simulink subsystem "bh_COMPONENT_model_7dof_car_SCAPE"  (R2022b)
settings: Solver=VariableStepAuto  StartTime=0.0  StopTime=10.0  RelTol=1e-3
model mask{L_b=0, L_f=0, L_R=0, L_L=0, m_c=0, I_cZ=0, I_cX=0, m_bR=0, m_fR=0, m_bL=0, m_fL=0, k_bR=0, k_fR=0, k_bL=0, k_fL=0, k_bRG=0, k_fRG=0, k_bLG=0, k_fLG=0, c_bR=0, c_fR=0, c_bL=0, c_fL=0, c_bRG=0, c_fRG=0, c_bLG=0, c_fLG=0, IC_pos=zeros(7,1), IC_vel=zeros(7,1)}
  mask prompts: L_b "L_b   (m)"; L_f "L_f   (m)"; L_R "L_R   (m)"; L_L "L_L   (m)"; m_c "m_c     (kg)"; I_cZ "I_cZ      (kg.m^2)"; I_cX "I_cX      (kg.m2)"; m_bR "m_bR   (kg)"; m_fR "m_fR    (kg)"; m_bL "m_bL   (kg)"; m_fL "m_fL    (kg)"; k_bR "k_bR   (N/m)"; k_fR "k_fR   (N/m)"; k_bL "k_bL   (N/m)"; k_fL "k_fL    (N/m)"; k_bRG "k_bRG   (N/m)"; k_fRG "k_fRG   (N/m)"; k_bLG "k_bLG   (N/m)"; k_fLG "k_fLG    (N/m)"; c_bR "c_bR  (N.s/m)"; c_fR "c_fR  (N.s/m)"; c_bL "c_bL  (N.s/m)"; c_fL "c_fL  (N.s/m)"; c_bRG "c_bRG  (N.s/m)"; c_fRG "c_fRG  (N.s/m)"; c_bLG "c_bLG  (N.s/m)"; c_fLG "c_fLG  (N.s/m)"
undefined symbols (not defined in the file): X, Y, Z
libraries: sm_lib x37, fl_lib x32, nesl_utility x14
settings Model: Creator=bhorton  LastModifiedBy=bhorton
settings DebuggingCC: UnconnectedInputMsg=warning  UnconnectedOutputMsg=warning  UnconnectedLineMsg=warning
settings ModelReferenceCC: EnableRefExpFcnMdlSchedulingChecks=on
settings RTWCC: DLArmComputeVersion=19.05

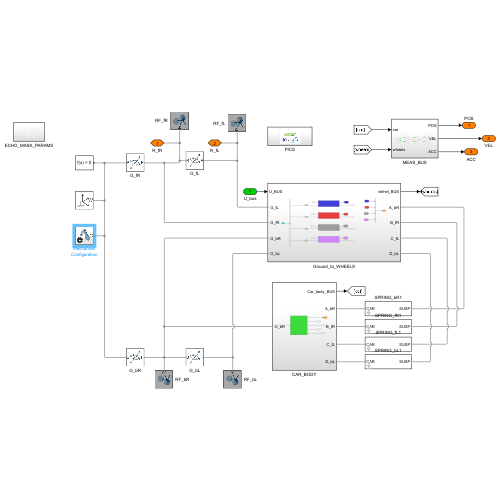
[thumbnail: Simulink's stored preview of the top-level diagram]
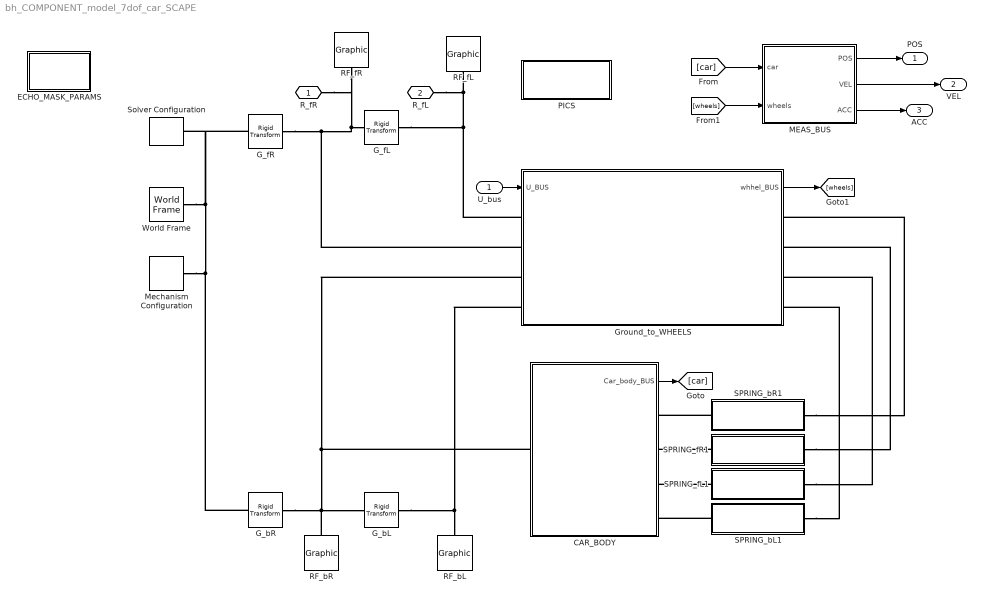
== system bh_COMPONENT_model_7dof_car_SCAPE ==
  U_bus : Inport
  CAR_BODY : Subsystem
  ECHO_MASK_PARAMS : Subsystem
  G_bL : sm_lib/Frames and Transforms/Rigid Transform  TranslationMethod=StandardAxis  TranslationStandardOffset=(L_L + L_R)  TranslationLengthUnit=m  TranslationStandardAxis=-Z  TranslationCartesianOffset=[0 0 0]  TranslationROffset=0  TranslationROffsetUnits=m  TranslationZOffset=0  TranslationZOffsetUnits=m  TranslationThetaOffset=0  TranslationThetaOffsetUnits=deg  RotationMethod=None  RotationAngleUnits=deg  RotationStandardAxis=+Z  RotationAngle=0.0  RotationArbitraryAxis=[0 0 1]  FollAlignAxisA=+X  BaseAlignAxisA=+Y  FollAlignAxisB=+Y  BaseAlignAxisB=+Z  RotationSequenceAxes=FollowerAxes  RotationSequence=XYX  RotationSequenceAngles=[0 0 0]  RotationSequenceAnglesUnits=deg  RotationMatrix=[1 0 0; 0 1 0; 0 0 1]  Quaternion=[1 0 0 0]
  G_bR : sm_lib/Frames and Transforms/Rigid Transform  TranslationMethod=None  TranslationStandardOffset=0  TranslationLengthUnit=m  TranslationStandardAxis=-X  TranslationCartesianOffset=[0 0 0]  TranslationROffset=0  TranslationROffsetUnits=m  TranslationZOffset=0  TranslationZOffsetUnits=m  TranslationThetaOffset=0  TranslationThetaOffsetUnits=deg  RotationMethod=None  RotationAngleUnits=deg  RotationStandardAxis=+Z  RotationAngle=0.0  RotationArbitraryAxis=[0 0 1]  FollAlignAxisA=+X  BaseAlignAxisA=+Y  FollAlignAxisB=+Y  BaseAlignAxisB=+Z  RotationSequenceAxes=FollowerAxes  RotationSequence=XYX  RotationSequenceAngles=[0 0 0]  RotationSequenceAnglesUnits=deg  RotationMatrix=[1 0 0; 0 1 0; 0 0 1]  Quaternion=[1 0 0 0]
  G_fL : sm_lib/Frames and Transforms/Rigid Transform  TranslationMethod=StandardAxis  TranslationStandardOffset=(L_L + L_R)  TranslationLengthUnit=m  TranslationStandardAxis=-Z  TranslationCartesianOffset=[0 0 0]  TranslationROffset=0  TranslationROffsetUnits=m  TranslationZOffset=0  TranslationZOffsetUnits=m  TranslationThetaOffset=0  TranslationThetaOffsetUnits=deg  RotationMethod=None  RotationAngleUnits=deg  RotationStandardAxis=+Z  RotationAngle=0.0  RotationArbitraryAxis=[0 0 1]  FollAlignAxisA=+X  BaseAlignAxisA=+Y  FollAlignAxisB=+Y  BaseAlignAxisB=+Z  RotationSequenceAxes=FollowerAxes  RotationSequence=XYX  RotationSequenceAngles=[0 0 0]  RotationSequenceAnglesUnits=deg  RotationMatrix=[1 0 0; 0 1 0; 0 0 1]  Quaternion=[1 0 0 0]
  G_fR : sm_lib/Frames and Transforms/Rigid Transform  TranslationMethod=StandardAxis  TranslationStandardOffset=(L_b + L_f)  TranslationLengthUnit=m  TranslationStandardAxis=+X  TranslationCartesianOffset=[0 0 0]  TranslationROffset=0  TranslationROffsetUnits=m  TranslationZOffset=0  TranslationZOffsetUnits=m  TranslationThetaOffset=0  TranslationThetaOffsetUnits=deg  RotationMethod=None  RotationAngleUnits=deg  RotationStandardAxis=+Z  RotationAngle=0.0  RotationArbitraryAxis=[0 0 1]  FollAlignAxisA=+X  BaseAlignAxisA=+Y  FollAlignAxisB=+Y  BaseAlignAxisB=+Z  RotationSequenceAxes=FollowerAxes  RotationSequence=XYX  RotationSequenceAngles=[0 0 0]  RotationSequenceAnglesUnits=deg  RotationMatrix=[1 0 0; 0 1 0; 0 0 1]  Quaternion=[1 0 0 0]
  Ground_to_WHEELS : Subsystem
  MEAS_BUS : Subsystem
  Mechanism Configuration : sm_lib/Utilities/Mechanism Configuration  UniformGravity=Constant  GravityVector=[0 0 0]  GravityUnits=m/s^2  LinearizationDelta=0.001  JointModeTransitionNonlinearIterations=2
  PICS : Subsystem
  RF_bL : sm_lib/Body Elements/Graphic  GraphicType=Marker  MarkerShape=Frame  MarkerSize=30  GraphicVisPropType=SimpleVisualProperties  GraphicDiffuseColor=[0.0 0.0 0.0]  GraphicSpecularColor=[0.5 0.5 0.5 1.0]  GraphicAmbientColor=[0.15 0.15 0.15 1.0]  GraphicEmissiveColor=[0.0 0.0 0.0 1.0]  GraphicShininess=75  GraphicOpacity=1.0
  RF_bR : sm_lib/Body Elements/Graphic  GraphicType=Marker  MarkerShape=Frame  MarkerSize=30  GraphicVisPropType=SimpleVisualProperties  GraphicDiffuseColor=[0.0 0.0 0.0]  GraphicSpecularColor=[0.5 0.5 0.5 1.0]  GraphicAmbientColor=[0.15 0.15 0.15 1.0]  GraphicEmissiveColor=[0.0 0.0 0.0 1.0]  GraphicShininess=75  GraphicOpacity=1.0
  RF_fL : sm_lib/Body Elements/Graphic  GraphicType=Marker  MarkerShape=Frame  MarkerSize=30  GraphicVisPropType=SimpleVisualProperties  GraphicDiffuseColor=[0.0 0.0 0.0]  GraphicSpecularColor=[0.5 0.5 0.5 1.0]  GraphicAmbientColor=[0.15 0.15 0.15 1.0]  GraphicEmissiveColor=[0.0 0.0 0.0 1.0]  GraphicShininess=75  GraphicOpacity=1.0
  RF_fR : sm_lib/Body Elements/Graphic  GraphicType=Marker  MarkerShape=Frame  MarkerSize=30  GraphicVisPropType=SimpleVisualProperties  GraphicDiffuseColor=[0.0 0.0 0.0]  GraphicSpecularColor=[0.5 0.5 0.5 1.0]  GraphicAmbientColor=[0.15 0.15 0.15 1.0]  GraphicEmissiveColor=[0.0 0.0 0.0 1.0]  GraphicShininess=75  GraphicOpacity=1.0
  SPRING_bL1 : Subsystem  mask{c=c_bL, k=k_bL, EQ_L=1}
  SPRING_bR1 : Subsystem  mask{c=c_bR, k=k_bR, EQ_L=1}
  SPRING_fL1 : Subsystem  mask{c=c_fL, k=k_fL, EQ_L=1}
  SPRING_fR1 : Subsystem  mask{c=c_fR, k=k_fR, EQ_L=1}
  Solver Configuration : nesl_utility/Solver Configuration  PhysicalDomain=network_engine_domain  SubClassName=solver  LeftPortType=input  RightPortType=generic  Tones=[]  Harmonics=[]  SimulateNoise=off  Profile=off  UseLocalSampling=off  EnableSwitchedLinearOptims=on  FrequencyDomain=off  UseCCode=off  RelTol=0.001  AbsTol=1e-06  MinStep=1e-09  ToWorkspace=off  RevertToSquareIcSolve=off  NumHomotopyIterations=100  PhasorMode=off  PhasorModeNumHarmonics=1  ConsistencySolver=NEWTON_FTOL  IndexReductionMethod=DerivativeReplacement  DoDC=off  ResidualTolerance=1e-09  ConsistencyTolSource=GLOBAL  ConsistencyAbsTol=0.001  ConsistencyRelTol=0.001  ConsistencyTolFactor=0.001  UseLocalSolver=off  LocalSolverChoice=NE_TRAPEZOIDAL_ADVANCER  ResolveIndetEquations=on  FunctionEvalNumThread=1  LocalSolverSampleTime=0.001  DoFixedCost=off  MaxNonlinIter=3  MaxModeIter=2  ComputeImpulses=off  ImpulseIterations=2  LinearAlgebra=Sparse  LinearAlgebraNumThread=0  EquationFormulation=NE_TIME_EF  DelaysMemoryBudget=1024  AutomaticFiltering=on  FilteringTimeConstant=0.001  PartitionStorageMethod=AS_NEEDED  PartitionMemoryBudget=1024  PartitionMethod=FAST
  World Frame : sm_lib/Frames and Transforms/World Frame
  R_fR : PMIOPort  Side=Left
  R_fL : PMIOPort  Port=2  Side=Left
  POS : Outport
  VEL : Outport  Port=2
  ACC : Outport  Port=3
  wires:
  MEAS_BUS/1(POS) -> POS/1
  MEAS_BUS/2(VEL) -> VEL/1
  MEAS_BUS/3(ACC) -> ACC/1
  U_bus/1 -> Ground_to_WHEELS/1(U_BUS)
  CAR_BODY/1(Car_body_BUS) -> [car]
  Ground_to_WHEELS/1(whhel_BUS) -> [wheels]
  [wheels] -> MEAS_BUS/2(wheels)
  [car] -> MEAS_BUS/1(car)
  connections:
  Mechanism Configuration/RConn1 -- G_bR/LConn1 -- G_fR/LConn1 -- Solver Configuration/RConn1 -- World Frame/RConn1
  G_bL/RConn1 -- RF_bL/RConn1 -- Ground_to_WHEELS/LConn4
  Ground_to_WHEELS/LConn3 -- RF_bR/RConn1 -- G_bL/LConn1 -- G_bR/RConn1 -- CAR_BODY/LConn1
  G_fL/RConn1 -- RF_fL/RConn1 -- R_fL/RConn1 -- Ground_to_WHEELS/LConn1
  Ground_to_WHEELS/LConn2 -- G_fL/LConn1 -- RF_fR/RConn1 -- R_fR/RConn1 -- G_fR/RConn1
  SPRING_bR1/RConn1 -- CAR_BODY/RConn1
  SPRING_fR1/RConn1 -- CAR_BODY/RConn2
  SPRING_fL1/RConn1 -- CAR_BODY/RConn3
  SPRING_bL1/RConn1 -- CAR_BODY/RConn4
  SPRING_bL1/LConn1 -- Ground_to_WHEELS/RConn4
  SPRING_fL1/LConn1 -- Ground_to_WHEELS/RConn3
  SPRING_fR1/LConn1 -- Ground_to_WHEELS/RConn2
  SPRING_bR1/LConn1 -- Ground_to_WHEELS/RConn1

== system bh_COMPONENT_model_7dof_car_SCAPE/CAR_BODY ==
  CAR_SYS : Subsystem  mask{m=m_c, I_X=I_cX, I_Z=I_cZ, EQ_L=1, init_pos_y=IC_pos(1), init_pos_pitch=IC_pos(2), init_pos_roll=IC_pos(3), init_vel_y=IC_vel(1), init_vel_pitch=IC_vel(2), init_vel_roll=IC_vel(3), L_b=L_b, L_f=L_f, L_R=L_R, L_L=L_L}
      mask init:
      | G_rel_to_R = bh_calc_G_rel_to_R(L_b, L_f, L_L, L_R);
      mask DialogControl Container6 Prompt: Inertia and ICs
      mask DialogControl Container18 Prompt: GEOM
  " G_bR" : PMIOPort  Side=Left
  A_bR : PMIOPort  Port=2  Side=Right
  B_fR : PMIOPort  Port=3  Side=Right
  C_fL : PMIOPort  Port=4  Side=Right
  D_bL : PMIOPort  Port=5  Side=Right
  Car_body_BUS : Outport
  wires:
  CAR_SYS/1(Car_body_BUS) -> Car_body_BUS/1
  connections:
  CAR_SYS/RConn4 -- D_bL/RConn1
  CAR_SYS/RConn3 -- C_fL/RConn1
  CAR_SYS/RConn2 -- B_fR/RConn1
  CAR_SYS/RConn1 -- A_bR/RConn1
  CAR_SYS/LConn1 -- " G_bR"/RConn1

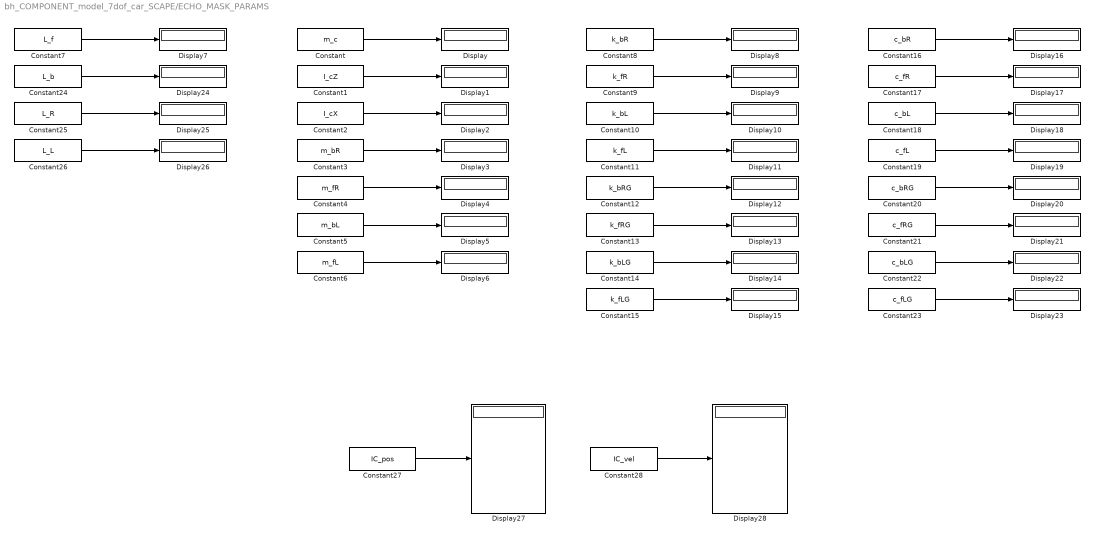
== system bh_COMPONENT_model_7dof_car_SCAPE/ECHO_MASK_PARAMS ==
  Constant : Constant  Value=m_c
  Constant1 : Constant  Value=I_cZ
  Constant10 : Constant  Value=k_bL
  Constant11 : Constant  Value=k_fL
  Constant12 : Constant  Value=k_bRG
  Constant13 : Constant  Value=k_fRG
  Constant14 : Constant  Value=k_bLG
  Constant15 : Constant  Value=k_fLG
  Constant16 : Constant  Value=c_bR
  Constant17 : Constant  Value=c_fR
  Constant18 : Constant  Value=c_bL
  Constant19 : Constant  Value=c_fL
  Constant2 : Constant  Value=I_cX
  Constant20 : Constant  Value=c_bRG
  Constant21 : Constant  Value=c_fRG
  Constant22 : Constant  Value=c_bLG
  Constant23 : Constant  Value=c_fLG
  Constant24 : Constant  Value=L_b
  Constant25 : Constant  Value=L_R
  Constant26 : Constant  Value=L_L
  Constant27 : Constant  Value=IC_pos
  Constant28 : Constant  Value=IC_vel
  Constant3 : Constant  Value=m_bR
  Constant4 : Constant  Value=m_fR
  Constant5 : Constant  Value=m_bL
  Constant6 : Constant  Value=m_fL
  Constant7 : Constant  Value=L_f
  Constant8 : Constant  Value=k_bR
  Constant9 : Constant  Value=k_fR
  Display{,1..28} (29 alike) : Display
  wires:
  Constant28/1 -> Display28/1
  Constant24/1 -> Display24/1
  Constant6/1 -> Display6/1
  Constant10/1 -> Display10/1
  Constant27/1 -> Display27/1
  Constant7/1 -> Display7/1
  Constant12/1 -> Display12/1
  Constant17/1 -> Display17/1
  Constant3/1 -> Display3/1
  Constant15/1 -> Display15/1
  Constant13/1 -> Display13/1
  Constant5/1 -> Display5/1
  Constant20/1 -> Display20/1
  Constant16/1 -> Display16/1
  Constant/1 -> Display/1
  Constant11/1 -> Display11/1
  Constant9/1 -> Display9/1
  Constant25/1 -> Display25/1
  Constant14/1 -> Display14/1
  Constant1/1 -> Display1/1
  Constant4/1 -> Display4/1
  Constant2/1 -> Display2/1
  Constant21/1 -> Display21/1
  Constant22/1 -> Display22/1
  Constant23/1 -> Display23/1
  Constant19/1 -> Display19/1
  Constant18/1 -> Display18/1
  Constant8/1 -> Display8/1
  Constant26/1 -> Display26/1

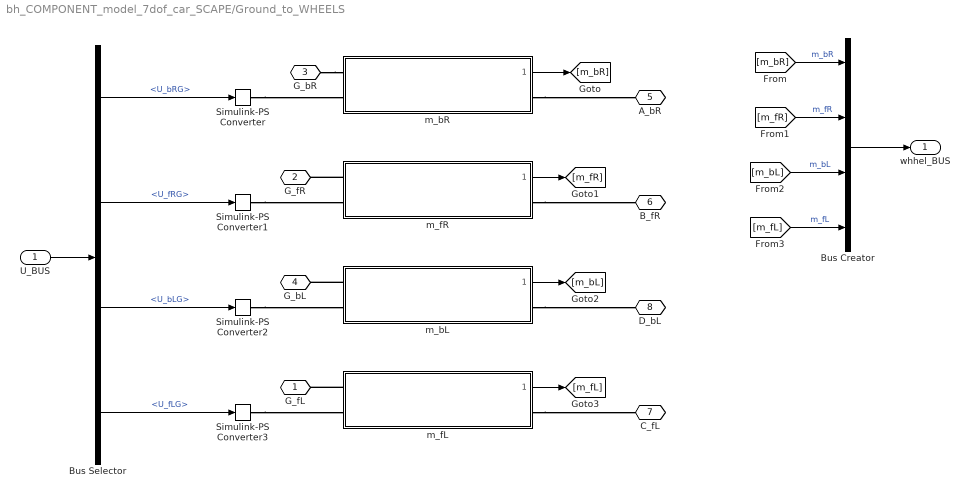
== system bh_COMPONENT_model_7dof_car_SCAPE/Ground_to_WHEELS ==
  U_BUS : Inport
  Bus Creator : BusCreator  Inputs=4
  Bus Selector : BusSelector  OutputSignals=U_bRG,U_fRG,U_bLG,U_fLG
  Simulink-PS Converter : nesl_utility/Simulink-PS Converter  PhysicalDomain=network_engine_domain  SubClassName=ps_input  LeftPortType=input  RightPortType=output  PseudoPeriodic=off  Frequencies=[]  NoiseDistribution=none  NoiseParameters=[]  Unit=m  AffineConversion=off  FilteringAndDerivatives=filter  SimscapeFilterOrder=2  InputFilterTimeConstant=1/5000  UdotUserProvided=1
  Simulink-PS Converter1 : nesl_utility/Simulink-PS Converter  PhysicalDomain=network_engine_domain  SubClassName=ps_input  LeftPortType=input  RightPortType=output  PseudoPeriodic=off  Frequencies=[]  NoiseDistribution=none  NoiseParameters=[]  Unit=m  AffineConversion=off  FilteringAndDerivatives=filter  SimscapeFilterOrder=2  InputFilterTimeConstant=1/5000  UdotUserProvided=0
  Simulink-PS Converter2 : nesl_utility/Simulink-PS Converter  PhysicalDomain=network_engine_domain  SubClassName=ps_input  LeftPortType=input  RightPortType=output  PseudoPeriodic=off  Frequencies=[]  NoiseDistribution=none  NoiseParameters=[]  Unit=m  AffineConversion=off  FilteringAndDerivatives=filter  SimscapeFilterOrder=2  InputFilterTimeConstant=1/5000  UdotUserProvided=0
  Simulink-PS Converter3 : nesl_utility/Simulink-PS Converter  PhysicalDomain=network_engine_domain  SubClassName=ps_input  LeftPortType=input  RightPortType=output  PseudoPeriodic=off  Frequencies=[]  NoiseDistribution=none  NoiseParameters=[]  Unit=m  AffineConversion=off  FilteringAndDerivatives=filter  SimscapeFilterOrder=2  InputFilterTimeConstant=1/5000  UdotUserProvided=0
  m_bL : Subsystem  ReferencedSubsystem=bh_COMPONENT_U_and_m  m_wheel=m_bL  c_G=c_bLG  k_G=k_bLG  EQ_L=1  y_wheel_init_pos=IC_pos(6)  y_wheel_init_vel=IC_vel(6)  Color=GREY
  m_bR : Subsystem  ReferencedSubsystem=bh_COMPONENT_U_and_m  m_wheel=m_bR  c_G=c_bRG  k_G=k_bRG  EQ_L=1  y_wheel_init_pos=IC_pos(4)  y_wheel_init_vel=IC_vel(4)  Color=BLUE
  m_fL : Subsystem  ReferencedSubsystem=bh_COMPONENT_U_and_m  m_wheel=m_fL  c_G=c_fLG  k_G=k_fLG  EQ_L=1  y_wheel_init_pos=IC_pos(7)  y_wheel_init_vel=IC_vel(7)  Color=PURPLE
  m_fR : Subsystem  ReferencedSubsystem=bh_COMPONENT_U_and_m  m_wheel=m_fR  c_G=c_fRG  k_G=k_fRG  EQ_L=1  y_wheel_init_pos=IC_pos(5)  y_wheel_init_vel=IC_vel(5)  Color=RED
  " G_fL" : PMIOPort  Side=Left
  " G_fR" : PMIOPort  Port=2  Side=Left
  " G_bR" : PMIOPort  Port=3  Side=Left
  " G_bL" : PMIOPort  Port=4  Side=Left
  A_bR : PMIOPort  Port=5  Side=Right
  B_fR : PMIOPort  Port=6  Side=Right
  C_fL : PMIOPort  Port=7  Side=Right
  D_bL : PMIOPort  Port=8  Side=Right
  whhel_BUS : Outport
  wires:
  [m_fL] -> Bus Creator/4  "m_fL"
  [m_bL] -> Bus Creator/3  "m_bL"
  [m_fR] -> Bus Creator/2  "m_fR"
  [m_bR] -> Bus Creator/1  "m_bR"
  m_bL/1 -> [m_bL]
  m_fR/1 -> [m_fR]
  m_bR/1 -> [m_bR]
  m_fL/1 -> [m_fL]
  Bus Creator/1 -> whhel_BUS/1
  Bus Selector/4 -> Simulink-PS Converter3/1  "<U_fLG>"
  Bus Selector/3 -> Simulink-PS Converter2/1  "<U_bLG>"
  Bus Selector/2 -> Simulink-PS Converter1/1  "<U_fRG>"
  Bus Selector/1 -> Simulink-PS Converter/1  "<U_bRG>"
  U_BUS/1 -> Bus Selector/1
  connections:
  Simulink-PS Converter3/RConn1 -- m_fL/LConn2
  Simulink-PS Converter2/RConn1 -- m_bL/LConn2
  Simulink-PS Converter1/RConn1 -- m_fR/LConn2
  Simulink-PS Converter/RConn1 -- m_bR/LConn2
  m_fL/RConn1 -- C_fL/RConn1
  m_fR/RConn1 -- B_fR/RConn1
  m_bL/RConn1 -- D_bL/RConn1
  m_bR/RConn1 -- A_bR/RConn1
  " G_bR"/RConn1 -- m_bR/LConn1
  m_bL/LConn1 -- " G_bL"/RConn1
  m_fL/LConn1 -- " G_fL"/RConn1
  m_fR/LConn1 -- " G_fR"/RConn1

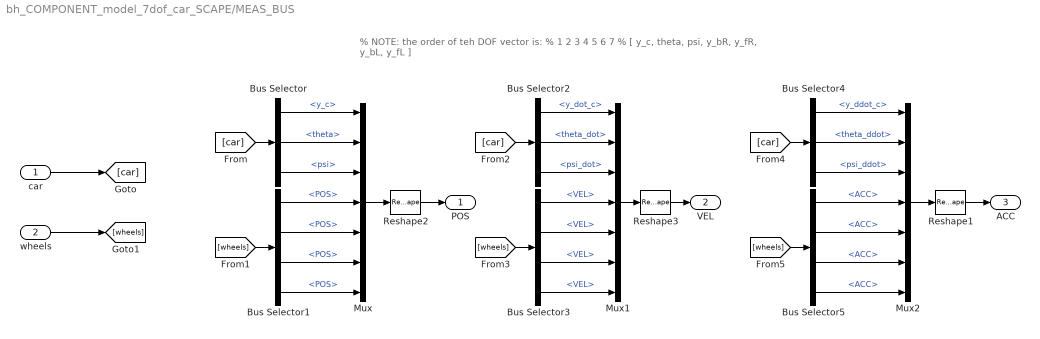
== system bh_COMPONENT_model_7dof_car_SCAPE/MEAS_BUS ==
  note: % NOTE:  the order of teh DOF vector is:
      | %          1      2    3     4     5     6     7
      | %      [ y_c, theta, psi, y_bR, y_fR, y_bL, y_fL ]
  car : Inport
  wheels : Inport  Port=2
  Bus Selector : BusSelector  OutputSignals=y_c.y_c,theta.theta,psi.psi
  Bus Selector1 : BusSelector  OutputSignals=m_bR.POS,m_fR.POS,m_bL.POS,m_fL.POS
  Bus Selector2 : BusSelector  OutputSignals=y_c.y_dot_c,theta.theta_dot,psi.psi_dot
  Bus Selector3 : BusSelector  OutputSignals=m_bR.VEL,m_fR.VEL,m_bL.VEL,m_fL.VEL
  Bus Selector4 : BusSelector  OutputSignals=y_c.y_ddot_c,theta.theta_ddot,psi.psi_ddot
  Bus Selector5 : BusSelector  OutputSignals=m_bR.ACC,m_fR.ACC,m_bL.ACC,m_fL.ACC
  Mux : Mux  Inputs=7
  Mux1 : Mux  Inputs=7
  Mux2 : Mux  Inputs=7
  Reshape1 : Reshape  OutputDimensionality=Column vector (2-D)
  Reshape2 : Reshape  OutputDimensionality=Column vector (2-D)
  Reshape3 : Reshape  OutputDimensionality=Column vector (2-D)
  POS : Outport
  VEL : Outport  Port=2
  ACC : Outport  Port=3
  wires:
  Reshape1/1 -> ACC/1
  Mux2/1 -> Reshape1/1
  Reshape3/1 -> VEL/1
  Reshape2/1 -> POS/1
  Mux/1 -> Reshape2/1
  Bus Selector5/1 -> Mux2/4  "<ACC>"
  Bus Selector5/2 -> Mux2/5  "<ACC>"
  [wheels] -> Bus Selector5/1
  Bus Selector4/2 -> Mux2/2  "<theta_ddot>"
  [car] -> Bus Selector4/1
  Bus Selector5/3 -> Mux2/6  "<ACC>"
  Bus Selector4/3 -> Mux2/3  "<psi_ddot>"
  Bus Selector4/1 -> Mux2/1  "<y_ddot_c>"
  Bus Selector5/4 -> Mux2/7  "<ACC>"
  Bus Selector3/4 -> Mux1/7  "<VEL>"
  Bus Selector2/3 -> Mux1/3  "<psi_dot>"
  Bus Selector2/1 -> Mux1/1  "<y_dot_c>"
  Bus Selector3/3 -> Mux1/6  "<VEL>"
  [wheels] -> Bus Selector3/1
  [car] -> Bus Selector2/1
  Mux1/1 -> Reshape3/1
  Bus Selector2/2 -> Mux1/2  "<theta_dot>"
  Bus Selector3/2 -> Mux1/5  "<VEL>"
  Bus Selector3/1 -> Mux1/4  "<VEL>"
  Bus Selector1/4 -> Mux/7  "<POS>"
  Bus Selector1/3 -> Mux/6  "<POS>"
  Bus Selector1/2 -> Mux/5  "<POS>"
  Bus Selector1/1 -> Mux/4  "<POS>"
  Bus Selector/3 -> Mux/3  "<psi>"
  Bus Selector/2 -> Mux/2  "<theta>"
  Bus Selector/1 -> Mux/1  "<y_c>"
  [wheels] -> Bus Selector1/1
  [car] -> Bus Selector/1
  car/1 -> [car]
  wheels/1 -> [wheels]

== system bh_COMPONENT_model_7dof_car_SCAPE/PICS ==

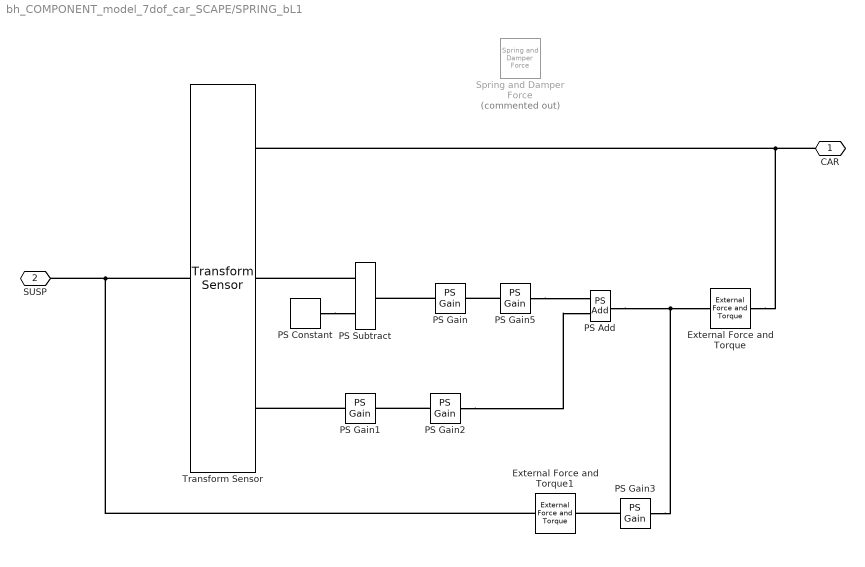
== system bh_COMPONENT_model_7dof_car_SCAPE/SPRING_bL1 ==
  External Force and Torque : sm_lib/Forces and Torques/External Force and Torque  ForceResolutionFrame=World  EnableForceX=off  EnableForceY=on  EnableForceZ=off  EnableForce=off  TorqueResolutionFrame=AttachedFrame  EnableTorqueX=off  EnableTorqueY=off  EnableTorqueZ=off  EnableTorque=off
  External Force and Torque1 : sm_lib/Forces and Torques/External Force and Torque  ForceResolutionFrame=World  EnableForceX=off  EnableForceY=on  EnableForceZ=off  EnableForce=off  TorqueResolutionFrame=AttachedFrame  EnableTorqueX=off  EnableTorqueY=off  EnableTorqueZ=off  EnableTorque=off
  PS Add : fl_lib/Physical Signals/Functions/PS Add
  PS Constant : fl_lib/Physical Signals/Sources/PS Constant  constant=EQ_L m
      settings: AttributesFormatString=%<constant> (%<constant_unit>)
  PS Gain : fl_lib/Physical Signals/Functions/PS Gain  gain=k N/m
      settings: AttributesFormatString=%<gain> (%<gain_unit>)
  PS Gain1 : fl_lib/Physical Signals/Functions/PS Gain  gain=c N*s/m
      settings: AttributesFormatString=%<gain> (%<gain_unit>)
  PS Gain2 : fl_lib/Physical Signals/Functions/PS Gain  gain=-1
      settings: AttributesFormatString=%<gain> (%<gain_unit>)
  PS Gain3 : fl_lib/Physical Signals/Functions/PS Gain  gain=-1
      settings: AttributesFormatString=%<gain> (%<gain_unit>)
  PS Gain5 : fl_lib/Physical Signals/Functions/PS Gain  gain=-1
      settings: AttributesFormatString=%<gain> (%<gain_unit>)
  PS Subtract : fl_lib/Physical Signals/Functions/PS Subtract
  Spring and Damper Force : sm_lib/Forces and Torques/Spring and Damper Force  Commented=on  NaturalLength=1  NaturalLengthUnits=m  SpringStiffness=100  SpringStiffnessUnits=N/m  DampingCoefficient=3  DampingCoefficientUnits=N/(m/s)  SenseForce=off
  Transform Sensor : sm_lib/Frames and Transforms/Transform Sensor  MeasurementFrame=World  SenseAngle=off  SenseAxis=off  SenseQ=off  SenseR=off  SenseRotationSequence=off  RotationSequence=XYX  SenseOmegaX=off  SenseOmegaY=off  SenseOmegaZ=off  SenseQDot=off  SenseRDot=off  SenseAlphaX=off  SenseAlphaY=off  SenseAlphaZ=off  SenseQDDot=off  SenseRDDot=off  SenseX=off  SenseY=on  SenseZ=off  SenseRad=off  SenseAzim=off  SenseDist=off  SenseInc=off  SenseXDot=off  SenseYDot=on  SenseZDot=off  SenseRadDot=off  SenseAzimDot=off  SenseDistDot=off  SenseIncDot=off  SenseXDDot=off  SenseYDDot=off  SenseZDDot=off  SenseRadDDot=off  SenseAzimDDot=off  SenseDistDDot=off  SenseIncDDot=off
  CAR : PMIOPort  Side=Right
  SUSP : PMIOPort  Port=2  Side=Left
  connections:
  PS Gain3/RConn1 -- External Force and Torque1/LConn1
  PS Gain3/LConn1 -- PS Add/RConn1 -- External Force and Torque/LConn1
  PS Gain2/RConn1 -- PS Add/LConn2
  PS Gain5/RConn1 -- PS Add/LConn1
  PS Gain2/LConn1 -- PS Gain1/RConn1
  PS Gain1/LConn1 -- Transform Sensor/RConn3
  PS Gain5/LConn1 -- PS Gain/RConn1
  PS Gain/LConn1 -- PS Subtract/RConn1
  PS Constant/RConn1 -- PS Subtract/LConn2
  PS Subtract/LConn1 -- Transform Sensor/RConn2
  External Force and Torque1/RConn1 -- Transform Sensor/LConn1 -- SUSP/RConn1
  CAR/RConn1 -- External Force and Torque/RConn1 -- Transform Sensor/RConn1

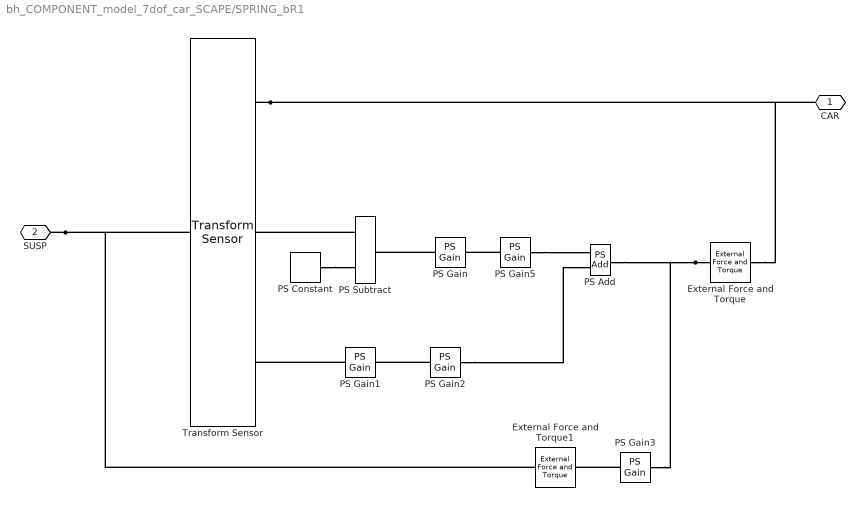
== system bh_COMPONENT_model_7dof_car_SCAPE/SPRING_bR1 ==
  External Force and Torque : sm_lib/Forces and Torques/External Force and Torque  ForceResolutionFrame=World  EnableForceX=off  EnableForceY=on  EnableForceZ=off  EnableForce=off  TorqueResolutionFrame=AttachedFrame  EnableTorqueX=off  EnableTorqueY=off  EnableTorqueZ=off  EnableTorque=off
  External Force and Torque1 : sm_lib/Forces and Torques/External Force and Torque  ForceResolutionFrame=World  EnableForceX=off  EnableForceY=on  EnableForceZ=off  EnableForce=off  TorqueResolutionFrame=AttachedFrame  EnableTorqueX=off  EnableTorqueY=off  EnableTorqueZ=off  EnableTorque=off
  PS Add : fl_lib/Physical Signals/Functions/PS Add
  PS Constant : fl_lib/Physical Signals/Sources/PS Constant  constant=EQ_L m
      settings: AttributesFormatString=%<constant> (%<constant_unit>)
  PS Gain : fl_lib/Physical Signals/Functions/PS Gain  gain=k N/m
      settings: AttributesFormatString=%<gain> (%<gain_unit>)
  PS Gain1 : fl_lib/Physical Signals/Functions/PS Gain  gain=c N*s/m
      settings: AttributesFormatString=%<gain> (%<gain_unit>)
  PS Gain2 : fl_lib/Physical Signals/Functions/PS Gain  gain=-1
      settings: AttributesFormatString=%<gain> (%<gain_unit>)
  PS Gain3 : fl_lib/Physical Signals/Functions/PS Gain  gain=-1
      settings: AttributesFormatString=%<gain> (%<gain_unit>)
  PS Gain5 : fl_lib/Physical Signals/Functions/PS Gain  gain=-1
      settings: AttributesFormatString=%<gain> (%<gain_unit>)
  PS Subtract : fl_lib/Physical Signals/Functions/PS Subtract
  Transform Sensor : sm_lib/Frames and Transforms/Transform Sensor  MeasurementFrame=World  SenseAngle=off  SenseAxis=off  SenseQ=off  SenseR=off  SenseRotationSequence=off  RotationSequence=XYX  SenseOmegaX=off  SenseOmegaY=off  SenseOmegaZ=off  SenseQDot=off  SenseRDot=off  SenseAlphaX=off  SenseAlphaY=off  SenseAlphaZ=off  SenseQDDot=off  SenseRDDot=off  SenseX=off  SenseY=on  SenseZ=off  SenseRad=off  SenseAzim=off  SenseDist=off  SenseInc=off  SenseXDot=off  SenseYDot=on  SenseZDot=off  SenseRadDot=off  SenseAzimDot=off  SenseDistDot=off  SenseIncDot=off  SenseXDDot=off  SenseYDDot=off  SenseZDDot=off  SenseRadDDot=off  SenseAzimDDot=off  SenseDistDDot=off  SenseIncDDot=off
  CAR : PMIOPort  Side=Right
  SUSP : PMIOPort  Port=2  Side=Left
  connections:
  PS Gain3/RConn1 -- External Force and Torque1/LConn1
  External Force and Torque/LConn1 -- PS Gain3/LConn1 -- PS Add/RConn1
  PS Gain2/RConn1 -- PS Add/LConn2
  PS Gain5/RConn1 -- PS Add/LConn1
  PS Gain2/LConn1 -- PS Gain1/RConn1
  PS Gain1/LConn1 -- Transform Sensor/RConn3
  PS Gain5/LConn1 -- PS Gain/RConn1
  PS Gain/LConn1 -- PS Subtract/RConn1
  PS Constant/RConn1 -- PS Subtract/LConn2
  PS Subtract/LConn1 -- Transform Sensor/RConn2
  SUSP/RConn1 -- External Force and Torque1/RConn1 -- Transform Sensor/LConn1
  Transform Sensor/RConn1 -- CAR/RConn1 -- External Force and Torque/RConn1

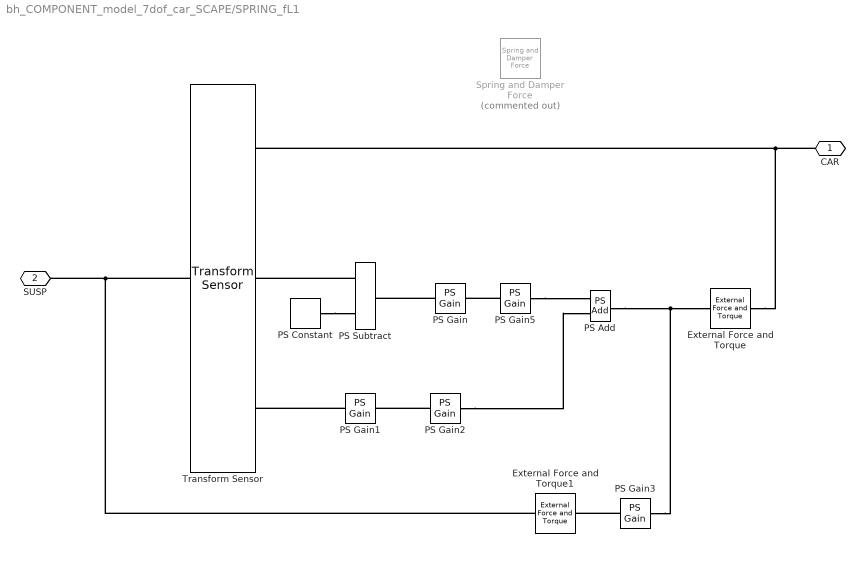
== system bh_COMPONENT_model_7dof_car_SCAPE/SPRING_fL1 ==
  External Force and Torque : sm_lib/Forces and Torques/External Force and Torque  ForceResolutionFrame=World  EnableForceX=off  EnableForceY=on  EnableForceZ=off  EnableForce=off  TorqueResolutionFrame=AttachedFrame  EnableTorqueX=off  EnableTorqueY=off  EnableTorqueZ=off  EnableTorque=off
  External Force and Torque1 : sm_lib/Forces and Torques/External Force and Torque  ForceResolutionFrame=World  EnableForceX=off  EnableForceY=on  EnableForceZ=off  EnableForce=off  TorqueResolutionFrame=AttachedFrame  EnableTorqueX=off  EnableTorqueY=off  EnableTorqueZ=off  EnableTorque=off
  PS Add : fl_lib/Physical Signals/Functions/PS Add
  PS Constant : fl_lib/Physical Signals/Sources/PS Constant  constant=EQ_L m
      settings: AttributesFormatString=%<constant> (%<constant_unit>)
  PS Gain : fl_lib/Physical Signals/Functions/PS Gain  gain=k N/m
      settings: AttributesFormatString=%<gain> (%<gain_unit>)
  PS Gain1 : fl_lib/Physical Signals/Functions/PS Gain  gain=c N*s/m
      settings: AttributesFormatString=%<gain> (%<gain_unit>)
  PS Gain2 : fl_lib/Physical Signals/Functions/PS Gain  gain=-1
      settings: AttributesFormatString=%<gain> (%<gain_unit>)
  PS Gain3 : fl_lib/Physical Signals/Functions/PS Gain  gain=-1
      settings: AttributesFormatString=%<gain> (%<gain_unit>)
  PS Gain5 : fl_lib/Physical Signals/Functions/PS Gain  gain=-1
      settings: AttributesFormatString=%<gain> (%<gain_unit>)
  PS Subtract : fl_lib/Physical Signals/Functions/PS Subtract
  Spring and Damper Force : sm_lib/Forces and Torques/Spring and Damper Force  Commented=on  NaturalLength=1  NaturalLengthUnits=m  SpringStiffness=100  SpringStiffnessUnits=N/m  DampingCoefficient=3  DampingCoefficientUnits=N/(m/s)  SenseForce=off
  Transform Sensor : sm_lib/Frames and Transforms/Transform Sensor  MeasurementFrame=World  SenseAngle=off  SenseAxis=off  SenseQ=off  SenseR=off  SenseRotationSequence=off  RotationSequence=XYX  SenseOmegaX=off  SenseOmegaY=off  SenseOmegaZ=off  SenseQDot=off  SenseRDot=off  SenseAlphaX=off  SenseAlphaY=off  SenseAlphaZ=off  SenseQDDot=off  SenseRDDot=off  SenseX=off  SenseY=on  SenseZ=off  SenseRad=off  SenseAzim=off  SenseDist=off  SenseInc=off  SenseXDot=off  SenseYDot=on  SenseZDot=off  SenseRadDot=off  SenseAzimDot=off  SenseDistDot=off  SenseIncDot=off  SenseXDDot=off  SenseYDDot=off  SenseZDDot=off  SenseRadDDot=off  SenseAzimDDot=off  SenseDistDDot=off  SenseIncDDot=off
  CAR : PMIOPort  Side=Right
  SUSP : PMIOPort  Port=2  Side=Left
  connections:
  PS Gain3/RConn1 -- External Force and Torque1/LConn1
  PS Gain3/LConn1 -- PS Add/RConn1 -- External Force and Torque/LConn1
  PS Gain2/RConn1 -- PS Add/LConn2
  PS Gain5/RConn1 -- PS Add/LConn1
  PS Gain2/LConn1 -- PS Gain1/RConn1
  PS Gain1/LConn1 -- Transform Sensor/RConn3
  PS Gain5/LConn1 -- PS Gain/RConn1
  PS Gain/LConn1 -- PS Subtract/RConn1
  PS Constant/RConn1 -- PS Subtract/LConn2
  PS Subtract/LConn1 -- Transform Sensor/RConn2
  External Force and Torque1/RConn1 -- Transform Sensor/LConn1 -- SUSP/RConn1
  CAR/RConn1 -- External Force and Torque/RConn1 -- Transform Sensor/RConn1

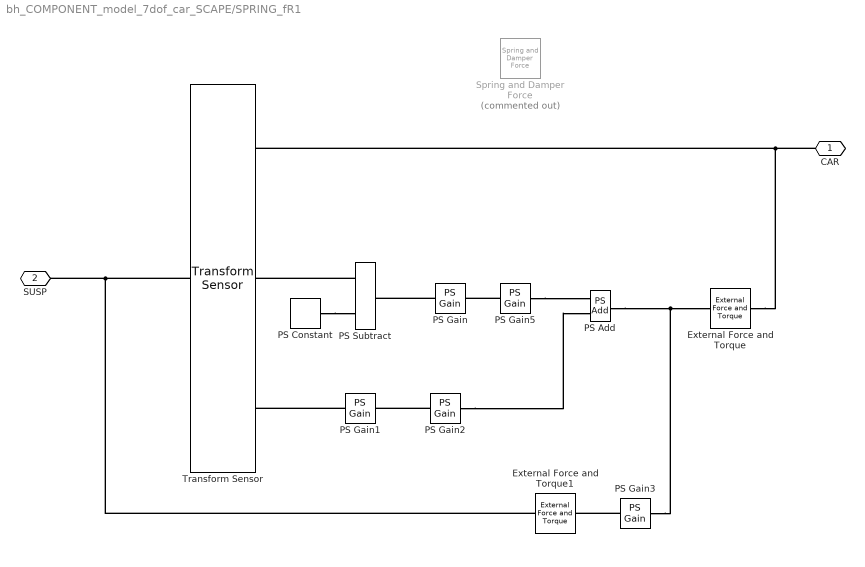
== system bh_COMPONENT_model_7dof_car_SCAPE/SPRING_fR1 ==
  External Force and Torque : sm_lib/Forces and Torques/External Force and Torque  ForceResolutionFrame=World  EnableForceX=off  EnableForceY=on  EnableForceZ=off  EnableForce=off  TorqueResolutionFrame=AttachedFrame  EnableTorqueX=off  EnableTorqueY=off  EnableTorqueZ=off  EnableTorque=off
  External Force and Torque1 : sm_lib/Forces and Torques/External Force and Torque  ForceResolutionFrame=World  EnableForceX=off  EnableForceY=on  EnableForceZ=off  EnableForce=off  TorqueResolutionFrame=AttachedFrame  EnableTorqueX=off  EnableTorqueY=off  EnableTorqueZ=off  EnableTorque=off
  PS Add : fl_lib/Physical Signals/Functions/PS Add
  PS Constant : fl_lib/Physical Signals/Sources/PS Constant  constant=EQ_L m
      settings: AttributesFormatString=%<constant> (%<constant_unit>)
  PS Gain : fl_lib/Physical Signals/Functions/PS Gain  gain=k N/m
      settings: AttributesFormatString=%<gain> (%<gain_unit>)
  PS Gain1 : fl_lib/Physical Signals/Functions/PS Gain  gain=c N*s/m
      settings: AttributesFormatString=%<gain> (%<gain_unit>)
  PS Gain2 : fl_lib/Physical Signals/Functions/PS Gain  gain=-1
      settings: AttributesFormatString=%<gain> (%<gain_unit>)
  PS Gain3 : fl_lib/Physical Signals/Functions/PS Gain  gain=-1
      settings: AttributesFormatString=%<gain> (%<gain_unit>)
  PS Gain5 : fl_lib/Physical Signals/Functions/PS Gain  gain=-1
      settings: AttributesFormatString=%<gain> (%<gain_unit>)
  PS Subtract : fl_lib/Physical Signals/Functions/PS Subtract
  Spring and Damper Force : sm_lib/Forces and Torques/Spring and Damper Force  Commented=on  NaturalLength=1  NaturalLengthUnits=m  SpringStiffness=100  SpringStiffnessUnits=N/m  DampingCoefficient=3  DampingCoefficientUnits=N/(m/s)  SenseForce=off
  Transform Sensor : sm_lib/Frames and Transforms/Transform Sensor  MeasurementFrame=World  SenseAngle=off  SenseAxis=off  SenseQ=off  SenseR=off  SenseRotationSequence=off  RotationSequence=XYX  SenseOmegaX=off  SenseOmegaY=off  SenseOmegaZ=off  SenseQDot=off  SenseRDot=off  SenseAlphaX=off  SenseAlphaY=off  SenseAlphaZ=off  SenseQDDot=off  SenseRDDot=off  SenseX=off  SenseY=on  SenseZ=off  SenseRad=off  SenseAzim=off  SenseDist=off  SenseInc=off  SenseXDot=off  SenseYDot=on  SenseZDot=off  SenseRadDot=off  SenseAzimDot=off  SenseDistDot=off  SenseIncDot=off  SenseXDDot=off  SenseYDDot=off  SenseZDDot=off  SenseRadDDot=off  SenseAzimDDot=off  SenseDistDDot=off  SenseIncDDot=off
  CAR : PMIOPort  Side=Right
  SUSP : PMIOPort  Port=2  Side=Left
  connections:
  PS Gain3/RConn1 -- External Force and Torque1/LConn1
  PS Gain3/LConn1 -- PS Add/RConn1 -- External Force and Torque/LConn1
  PS Gain2/RConn1 -- PS Add/LConn2
  PS Gain5/RConn1 -- PS Add/LConn1
  PS Gain2/LConn1 -- PS Gain1/RConn1
  PS Gain1/LConn1 -- Transform Sensor/RConn3
  PS Gain5/LConn1 -- PS Gain/RConn1
  PS Gain/LConn1 -- PS Subtract/RConn1
  PS Constant/RConn1 -- PS Subtract/LConn2
  PS Subtract/LConn1 -- Transform Sensor/RConn2
  External Force and Torque1/RConn1 -- Transform Sensor/LConn1 -- SUSP/RConn1
  CAR/RConn1 -- External Force and Torque/RConn1 -- Transform Sensor/RConn1

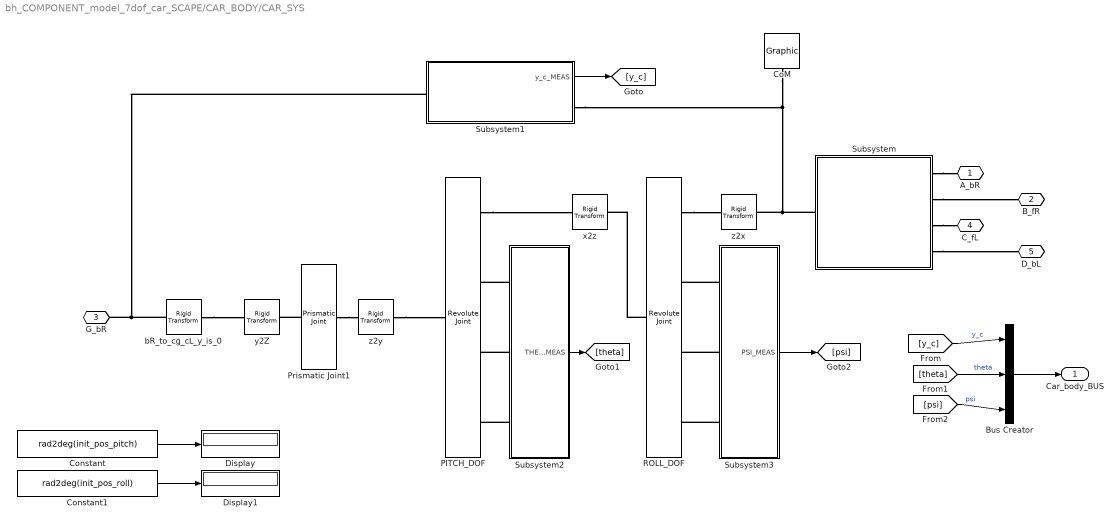
== system bh_COMPONENT_model_7dof_car_SCAPE/CAR_BODY/CAR_SYS ==
  Bus Creator : BusCreator  Inputs=3
  CoM : sm_lib/Body Elements/Graphic  GraphicType=Marker  MarkerShape=Frame  MarkerSize=30  GraphicVisPropType=SimpleVisualProperties  GraphicDiffuseColor=[0.0 0.0 0.0]  GraphicSpecularColor=[0.5 0.5 0.5 1.0]  GraphicAmbientColor=[0.15 0.15 0.15 1.0]  GraphicEmissiveColor=[0.0 0.0 0.0 1.0]  GraphicShininess=75  GraphicOpacity=1.0
  Constant : Constant  Value=rad2deg(init_pos_pitch)
  Constant1 : Constant  Value=rad2deg(init_pos_roll)
  Display : Display
  Display1 : Display
  PITCH_DOF : sm_lib/Joints/Revolute Joint  JointMode=Normal  SenseConstraintForce=off  SenseConstraintForceX=off  SenseConstraintForceY=off  SenseConstraintForceZ=off  SenseConstraintTorque=off  SenseConstraintTorqueX=off  SenseConstraintTorqueY=off  SenseConstraintTorqueZ=off  SenseTotalForce=off  SenseTotalForceX=off  SenseTotalForceY=off  SenseTotalForceZ=off  SenseTotalTorque=off  SenseTotalTorqueX=off  SenseTotalTorqueY=off  SenseTotalTorqueZ=off  CompositeWrenchDir=FollowerOnBase  CompositeWrenchFrame=BaseFrame  EquilibriumPosition=0  EquilibriumPositionUnits=deg  SpringStiffness=0  SpringStiffnessUnits=N*m/deg  DampingCoefficient=0  DampingCoefficientUnits=N*m/(deg/s)  TorqueActuationMode=NoTorque  MotionActuationMode=ComputedMotion  SensePosition=on  SenseVelocity=on  SenseAcceleration=on  SenseTorqueForce=off  SenseLowerLimitTorqueForce=off  SenseUpperLimitTorqueForce=off  LowerLimitSpecify=off  LowerLimitBound=-90  LowerLimitBoundUnits=deg  LowerLimitStiffness=1e4  LowerLimitStiffnessUnits=N*m/deg  LowerLimitDamping=10  LowerLimitDampingUnits=N*m/(deg/s)  LowerLimitTransitionRegionWidth=0.1  LowerLimitTransitionRegionWidthUnits=deg  UpperLimitSpecify=off  UpperLimitBound=90  UpperLimitBoundUnits=deg  UpperLimitStiffness=1e4  UpperLimitStiffnessUnits=N*m/deg  UpperLimitDamping=10  UpperLimitDampingUnits=N*m/(deg/s)  UpperLimitTransitionRegionWidth=0.1  UpperLimitTransitionRegionWidthUnits=deg  PositionTargetSpecify=on  PositionTargetPriority=High  PositionTargetValue=init_pos_pitch  PositionTargetValueUnits=rad  VelocityTargetSpecify=on  VelocityTargetPriority=High  VelocityTargetValue=init_vel_pitch  VelocityTargetValueUnits=rad/s
      settings: AttributesFormatString=|
      | IC_POS =%<PositionTargetValue> (%<PositionTargetValueUnits>)
      | IC_VEL = %<VelocityTargetValue> (%<VelocityTargetValueUnits>)
  Prismatic Joint1 : sm_lib/Joints/Prismatic Joint  JointMode=Normal  SenseConstraintForce=off  SenseConstraintForceX=off  SenseConstraintForceY=off  SenseConstraintForceZ=off  SenseConstraintTorque=off  SenseConstraintTorqueX=off  SenseConstraintTorqueY=off  SenseConstraintTorqueZ=off  SenseTotalForce=off  SenseTotalForceX=off  SenseTotalForceY=off  SenseTotalForceZ=off  SenseTotalTorque=off  SenseTotalTorqueX=off  SenseTotalTorqueY=off  SenseTotalTorqueZ=off  CompositeWrenchDir=FollowerOnBase  CompositeWrenchFrame=BaseFrame  EquilibriumPosition=0  EquilibriumPositionUnits=m  SpringStiffness=0  SpringStiffnessUnits=N/m  DampingCoefficient=0  DampingCoefficientUnits=N/(m/s)  TorqueActuationMode=NoTorque  MotionActuationMode=ComputedMotion  SensePosition=off  SenseVelocity=off  SenseAcceleration=off  SenseTorqueForce=off  SenseLowerLimitTorqueForce=off  SenseUpperLimitTorqueForce=off  LowerLimitSpecify=off  LowerLimitBound=-1  LowerLimitBoundUnits=m  LowerLimitStiffness=1e6  LowerLimitStiffnessUnits=N/m  LowerLimitDamping=1e3  LowerLimitDampingUnits=N/(m/s)  LowerLimitTransitionRegionWidth=1e-4  LowerLimitTransitionRegionWidthUnits=m  UpperLimitSpecify=off  UpperLimitBound=1  UpperLimitBoundUnits=m  UpperLimitStiffness=1e6  UpperLimitStiffnessUnits=N/m  UpperLimitDamping=1e3  UpperLimitDampingUnits=N/(m/s)  UpperLimitTransitionRegionWidth=1e-4  UpperLimitTransitionRegionWidthUnits=m  PositionTargetSpecify=on  PositionTargetPriority=High  PositionTargetValue=init_pos_y + 2*EQ_L  PositionTargetValueUnits=m  VelocityTargetSpecify=on  VelocityTargetPriority=High  VelocityTargetValue=init_vel_y  VelocityTargetValueUnits=m/s
      settings: AttributesFormatString=|
      | vel = %<VelocityTargetValue> (%<VelocityTargetValueUnits>)
      | pos = %<PositionTargetValue> (%<PositionTargetValueUnits>)
  ROLL_DOF : sm_lib/Joints/Revolute Joint  JointMode=Normal  SenseConstraintForce=off  SenseConstraintForceX=off  SenseConstraintForceY=off  SenseConstraintForceZ=off  SenseConstraintTorque=off  SenseConstraintTorqueX=off  SenseConstraintTorqueY=off  SenseConstraintTorqueZ=off  SenseTotalForce=off  SenseTotalForceX=off  SenseTotalForceY=off  SenseTotalForceZ=off  SenseTotalTorque=off  SenseTotalTorqueX=off  SenseTotalTorqueY=off  SenseTotalTorqueZ=off  CompositeWrenchDir=FollowerOnBase  CompositeWrenchFrame=BaseFrame  EquilibriumPosition=0  EquilibriumPositionUnits=deg  SpringStiffness=0  SpringStiffnessUnits=N*m/deg  DampingCoefficient=0  DampingCoefficientUnits=N*m/(deg/s)  TorqueActuationMode=NoTorque  MotionActuationMode=ComputedMotion  SensePosition=on  SenseVelocity=on  SenseAcceleration=on  SenseTorqueForce=off  SenseLowerLimitTorqueForce=off  SenseUpperLimitTorqueForce=off  LowerLimitSpecify=off  LowerLimitBound=-90  LowerLimitBoundUnits=deg  LowerLimitStiffness=1e4  LowerLimitStiffnessUnits=N*m/deg  LowerLimitDamping=10  LowerLimitDampingUnits=N*m/(deg/s)  LowerLimitTransitionRegionWidth=0.1  LowerLimitTransitionRegionWidthUnits=deg  UpperLimitSpecify=off  UpperLimitBound=90  UpperLimitBoundUnits=deg  UpperLimitStiffness=1e4  UpperLimitStiffnessUnits=N*m/deg  UpperLimitDamping=10  UpperLimitDampingUnits=N*m/(deg/s)  UpperLimitTransitionRegionWidth=0.1  UpperLimitTransitionRegionWidthUnits=deg  PositionTargetSpecify=on  PositionTargetPriority=High  PositionTargetValue=init_pos_roll  PositionTargetValueUnits=rad  VelocityTargetSpecify=on  VelocityTargetPriority=High  VelocityTargetValue=init_vel_roll  VelocityTargetValueUnits=rad/s
      settings: AttributesFormatString=|
      | IC_POS =%<PositionTargetValue> (%<PositionTargetValueUnits>)
      | IC_VEL = %<VelocityTargetValue> (%<VelocityTargetValueUnits>)
  Subsystem : Subsystem
  Subsystem1 : Subsystem
  Subsystem2 : Subsystem
  Subsystem3 : Subsystem
  bR_to_cg_cL_y_is_0 : sm_lib/Frames and Transforms/Rigid Transform  TranslationMethod=Cartesian  TranslationStandardOffset=(L_L + L_R)  TranslationLengthUnit=m  TranslationStandardAxis=-Z  TranslationCartesianOffset=[L_b, 0, (-L_R)]  TranslationROffset=0  TranslationROffsetUnits=m  TranslationZOffset=0  TranslationZOffsetUnits=m  TranslationThetaOffset=0  TranslationThetaOffsetUnits=deg  RotationMethod=None  RotationAngleUnits=deg  RotationStandardAxis=+Z  RotationAngle=0.0  RotationArbitraryAxis=[0 0 1]  FollAlignAxisA=+X  BaseAlignAxisA=+Y  FollAlignAxisB=+Y  BaseAlignAxisB=+Z  RotationSequenceAxes=FollowerAxes  RotationSequence=XYX  RotationSequenceAngles=[0 0 0]  RotationSequenceAnglesUnits=deg  RotationMatrix=[1 0 0; 0 1 0; 0 0 1]  Quaternion=[1 0 0 0]
  x2z : sm_lib/Frames and Transforms/Rigid Transform  TranslationMethod=None  TranslationStandardOffset=0  TranslationLengthUnit=m  TranslationStandardAxis=+Z  TranslationCartesianOffset=[0 0 0]  TranslationROffset=0  TranslationROffsetUnits=m  TranslationZOffset=0  TranslationZOffsetUnits=m  TranslationThetaOffset=0  TranslationThetaOffsetUnits=deg  RotationMethod=AlignedAxes  RotationAngleUnits=deg  RotationStandardAxis=+Z  RotationAngle=0.0  RotationArbitraryAxis=[0 0 1]  FollAlignAxisA=+Z  BaseAlignAxisA=+X  FollAlignAxisB=+Y  BaseAlignAxisB=+Y  RotationSequenceAxes=FollowerAxes  RotationSequence=XYX  RotationSequenceAngles=[0 0 0]  RotationSequenceAnglesUnits=deg  RotationMatrix=[1 0 0; 0 1 0; 0 0 1]  Quaternion=[1 0 0 0]
  y2Z : sm_lib/Frames and Transforms/Rigid Transform  TranslationMethod=None  TranslationStandardOffset=0  TranslationLengthUnit=m  TranslationStandardAxis=+Z  TranslationCartesianOffset=[0 0 0]  TranslationROffset=0  TranslationROffsetUnits=m  TranslationZOffset=0  TranslationZOffsetUnits=m  TranslationThetaOffset=0  TranslationThetaOffsetUnits=deg  RotationMethod=AlignedAxes  RotationAngleUnits=deg  RotationStandardAxis=+Z  RotationAngle=0.0  RotationArbitraryAxis=[0 0 1]  FollAlignAxisA=+Z  BaseAlignAxisA=+Y  FollAlignAxisB=+X  BaseAlignAxisB=+X  RotationSequenceAxes=FollowerAxes  RotationSequence=XYX  RotationSequenceAngles=[0 0 0]  RotationSequenceAnglesUnits=deg  RotationMatrix=[1 0 0; 0 1 0; 0 0 1]  Quaternion=[1 0 0 0]
  z2x : sm_lib/Frames and Transforms/Rigid Transform  TranslationMethod=None  TranslationStandardOffset=0  TranslationLengthUnit=m  TranslationStandardAxis=+Z  TranslationCartesianOffset=[0 0 0]  TranslationROffset=0  TranslationROffsetUnits=m  TranslationZOffset=0  TranslationZOffsetUnits=m  TranslationThetaOffset=0  TranslationThetaOffsetUnits=deg  RotationMethod=AlignedAxes  RotationAngleUnits=deg  RotationStandardAxis=+Z  RotationAngle=0.0  RotationArbitraryAxis=[0 0 1]  FollAlignAxisA=+X  BaseAlignAxisA=+Z  FollAlignAxisB=+Y  BaseAlignAxisB=+Y  RotationSequenceAxes=FollowerAxes  RotationSequence=XYX  RotationSequenceAngles=[0 0 0]  RotationSequenceAnglesUnits=deg  RotationMatrix=[1 0 0; 0 1 0; 0 0 1]  Quaternion=[1 0 0 0]
  z2y : sm_lib/Frames and Transforms/Rigid Transform  TranslationMethod=None  TranslationStandardOffset=0  TranslationLengthUnit=m  TranslationStandardAxis=+Z  TranslationCartesianOffset=[0 0 0]  TranslationROffset=0  TranslationROffsetUnits=m  TranslationZOffset=0  TranslationZOffsetUnits=m  TranslationThetaOffset=0  TranslationThetaOffsetUnits=deg  RotationMethod=AlignedAxes  RotationAngleUnits=deg  RotationStandardAxis=+Z  RotationAngle=0.0  RotationArbitraryAxis=[0 0 1]  FollAlignAxisA=+Y  BaseAlignAxisA=+Z  FollAlignAxisB=+X  BaseAlignAxisB=+X  RotationSequenceAxes=FollowerAxes  RotationSequence=XYX  RotationSequenceAngles=[0 0 0]  RotationSequenceAnglesUnits=deg  RotationMatrix=[1 0 0; 0 1 0; 0 0 1]  Quaternion=[1 0 0 0]
  A_bR : PMIOPort  Side=Right
  B_fR : PMIOPort  Port=2  Side=Right
  G_bR : PMIOPort  Port=3  Side=Left
  C_fL : PMIOPort  Port=4  Side=Right
  D_bL : PMIOPort  Port=5  Side=Right
  Car_body_BUS : Outport
  wires:
  Bus Creator/1 -> Car_body_BUS/1
  [y_c] -> Bus Creator/1  "y_c"
  [theta] -> Bus Creator/2  "theta"
  [psi] -> Bus Creator/3  "psi"
  Subsystem3/1(PSI_MEAS) -> [psi]
  Subsystem2/1(THETA_MEAS) -> [theta]
  Subsystem1/1(y_c_MEAS) -> [y_c]
  Constant1/1 -> Display1/1
  Constant/1 -> Display/1
  connections:
  Subsystem3/LConn3 -- ROLL_DOF/RConn4
  Subsystem3/LConn2 -- ROLL_DOF/RConn3
  Subsystem3/LConn1 -- ROLL_DOF/RConn2
  Subsystem2/LConn1 -- PITCH_DOF/RConn2
  Subsystem2/LConn3 -- PITCH_DOF/RConn4
  Subsystem2/LConn2 -- PITCH_DOF/RConn3
  ROLL_DOF/RConn1 -- z2x/LConn1
  Prismatic Joint1/LConn1 -- y2Z/RConn1
  Subsystem/LConn2 -- B_fR/RConn1
  ROLL_DOF/LConn1 -- x2z/RConn1
  PITCH_DOF/RConn1 -- x2z/LConn1
  Subsystem/LConn4 -- D_bL/RConn1
  Prismatic Joint1/RConn1 -- z2y/LConn1
  z2y/RConn1 -- PITCH_DOF/LConn1
  bR_to_cg_cL_y_is_0/RConn1 -- y2Z/LConn1
  Subsystem/LConn1 -- A_bR/RConn1
  Subsystem1/RConn1 -- CoM/RConn1 -- z2x/RConn1 -- Subsystem/RConn1
  Subsystem/LConn3 -- C_fL/RConn1
  bR_to_cg_cL_y_is_0/LConn1 -- Subsystem1/LConn1 -- G_bR/RConn1

== system bh_COMPONENT_model_7dof_car_SCAPE/CAR_BODY/CAR_SYS/Subsystem ==
  " CAR" : sm_lib/Body Elements/Brick Solid  GraphicAmbientColor=[0.15 0.15 0.15 1.0]  BasedOnType=Density  BrickDimensions=[(L_b+L_f), 0.25, (L_R+L_L)]  BrickDimensionUnits=m  CenterOfMass=G_rel_to_R  CenterOfMassUnits=m  GraphicDiffuseColor=[0.0 1.0 0.2]  Density=1000  DensityUnits=kg/m^3  DoExposeReferenceFrame=on  GraphicEmissiveColor=[0.0 0.0 0.0 1.0]  ExportEntireGeometry=off  SerializedFrames=<Frames><Frame><Id>Frame1</Id><Value><Name>A</Name><Origin><Source>GeometricFeature</Source><FeatureName>+z -x curve</FeatureName></Origin><PrimaryAxis><DefinedDirection>+Z</DefinedDirection><Source>ReferenceFrame</Source><SourceDirection>+Z</SourceDirection><FeatureName></FeatureName></PrimaryAxis><SecondaryAxis><DefinedDirection>+X</DefinedDirection><Source>ReferenceFrame</Source><SourceDirection>+X</SourceDirection><FeatureName></FeatureName></SecondaryAxis></Value></Frame><Frame><Id>Frame2</Id><Value><Name>B</Name><Origin><Source>GeometricFeature</Source><FeatureName>+z +x curve</FeatureName></Origin><PrimaryAxis><DefinedDirection>+Z</DefinedDirection><Source>ReferenceFrame</Source><SourceDirection>+Z</SourceDirection><FeatureName></FeatureName></PrimaryAxis><SecondaryAxis><DefinedDirection>+X</DefinedDirection><Source>ReferenceFrame</Source><SourceDirection>+X</SourceDirection><FeatureName></FeatureName></SecondaryAxis></Value></Frame><Frame><Id>Frame3</Id><Value><Name>C</Name><Origin><Source>GeometricFeature</Source><FeatureName>-z +x curve</FeatureName></Origin><PrimaryAxis><DefinedDirection>+Z</DefinedDirection><Source>ReferenceFrame</Source><SourceDirection>+Z</SourceDirection><FeatureName></FeatureName></PrimaryAxis><SecondaryAxis><DefinedDirection>+X</DefinedDirection><Source>ReferenceFrame</Source><SourceDirection>+X</SourceDirection><FeatureName></FeatureName></SecondaryAxis></Value></Frame><Frame><Id>Frame4</Id><Value><Name>D</Name><Origin><Source>GeometricFeature</Source><FeatureName>-z -x curve</FeatureName></Origin><PrimaryAxis><DefinedDirection>+Z</DefinedDirection><Source>ReferenceFrame</Source><SourceDirection>+Z</SourceDirection><FeatureName></FeatureName></PrimaryAxis><SecondaryAxis><DefinedDirection>+X</DefinedDirection><Source>ReferenceFrame</Source><SourceDirection>+X</SourceDirection><FeatureName></FeatureName></SecondaryAxis></Value></Frame><Frame><Id>Frame5</Id><Value><Name>CoM</Name><Origin><Source>CenterOfMassFrame</Source><FeatureName></FeatureName></Origin><PrimaryAxis><DefinedDirection>+Z</DefinedDirection><Source>ReferenceFrame</Source><SourceDirection>+Z</SourceDirection><FeatureName></FeatureName></PrimaryAxis><SecondaryAxis><DefinedDirection>+X</DefinedDirection><Source>ReferenceFrame</Source><SourceDirection>+X</SourceDirection><FeatureName></FeatureName></SecondaryAxis></Value></Frame></Frames>  MarkerShape=Sphere  MarkerSize=10  GraphicType=FromGeometry  InertiaType=Custom  Mass=m  MassUnits=kg  MomentsOfInertia="[I_X ,  5*I_X ,  I_Z]"  MomentsOfInertiaUnits=kg*m^2  GraphicOpacity=1.0  ProductsOfInertia=[0 0 0]  ProductsOfInertiaUnits=kg*m^2  GraphicShininess=75  GraphicSpecularColor=[0.5 0.5 0.5 1.0]  GraphicVisPropType=SimpleVisualProperties
  R : sm_lib/Body Elements/Graphic  Commented=on  GraphicType=Marker  MarkerShape=Frame  MarkerSize=30  GraphicVisPropType=SimpleVisualProperties  GraphicDiffuseColor=[0.0 0.2 1.0]  GraphicSpecularColor=[0.5 0.5 0.5 1.0]  GraphicAmbientColor=[0.15 0.15 0.15 1.0]  GraphicEmissiveColor=[0.0 0.0 0.0 1.0]  GraphicShininess=75  GraphicOpacity=1.0
  A : PMIOPort  Side=Left
  B : PMIOPort  Port=2  Side=Left
  C : PMIOPort  Port=3  Side=Left
  D : PMIOPort  Port=4  Side=Left
  COM : PMIOPort  Port=5  Side=Right
  connections:
  R/RConn1 -- " CAR"/RConn1
  " CAR"/LConn1 -- A/RConn1
  " CAR"/LConn3 -- D/RConn1
  " CAR"/RConn3 -- COM/RConn1
  " CAR"/RConn2 -- C/RConn1
  " CAR"/LConn2 -- B/RConn1

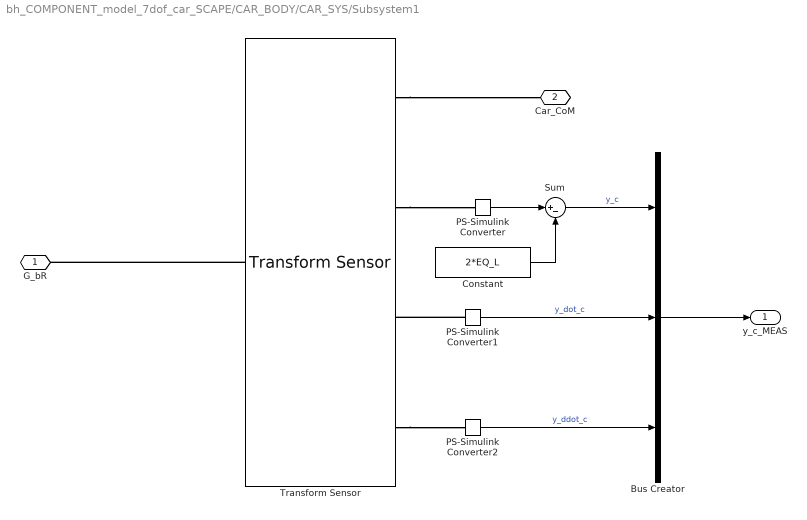
== system bh_COMPONENT_model_7dof_car_SCAPE/CAR_BODY/CAR_SYS/Subsystem1 ==
  Bus Creator : BusCreator  Inputs=3
  Constant : Constant  Value=2*EQ_L
  PS-Simulink Converter : nesl_utility/PS-Simulink Converter  PhysicalDomain=network_engine_domain  SubClassName=ps_output  LeftPortType=input  RightPortType=output  PseudoPeriodic=off  Frequencies=[]  VectorFormat=1-D array  Unit=m  AffineConversion=off
  PS-Simulink Converter1 : nesl_utility/PS-Simulink Converter  PhysicalDomain=network_engine_domain  SubClassName=ps_output  LeftPortType=input  RightPortType=output  PseudoPeriodic=off  Frequencies=[]  VectorFormat=1-D array  Unit=m/s  AffineConversion=off
  PS-Simulink Converter2 : nesl_utility/PS-Simulink Converter  PhysicalDomain=network_engine_domain  SubClassName=ps_output  LeftPortType=input  RightPortType=output  PseudoPeriodic=off  Frequencies=[]  VectorFormat=1-D array  Unit=m/s^2  AffineConversion=off
  Sum : Sum  Inputs=|+-
  Transform Sensor : sm_lib/Frames and Transforms/Transform Sensor  MeasurementFrame=World  SenseAngle=off  SenseAxis=off  SenseQ=off  SenseR=off  SenseRotationSequence=off  RotationSequence=XYX  SenseOmegaX=off  SenseOmegaY=off  SenseOmegaZ=off  SenseQDot=off  SenseRDot=off  SenseAlphaX=off  SenseAlphaY=off  SenseAlphaZ=off  SenseQDDot=off  SenseRDDot=off  SenseX=off  SenseY=on  SenseZ=off  SenseRad=off  SenseAzim=off  SenseDist=off  SenseInc=off  SenseXDot=off  SenseYDot=on  SenseZDot=off  SenseRadDot=off  SenseAzimDot=off  SenseDistDot=off  SenseIncDot=off  SenseXDDot=off  SenseYDDot=on  SenseZDDot=off  SenseRadDDot=off  SenseAzimDDot=off  SenseDistDDot=off  SenseIncDDot=off
  G_bR : PMIOPort  Side=Left
  Car_CoM : PMIOPort  Port=2  Side=Right
  y_c_MEAS : Outport
  wires:
  Bus Creator/1 -> y_c_MEAS/1
  PS-Simulink Converter2/1 -> Bus Creator/3  "y_ddot_c"
  PS-Simulink Converter1/1 -> Bus Creator/2  "y_dot_c"
  Sum/1 -> Bus Creator/1  "y_c"
  Constant/1 -> Sum/2
  PS-Simulink Converter/1 -> Sum/1
  connections:
  Transform Sensor/RConn4 -- PS-Simulink Converter2/LConn1
  PS-Simulink Converter1/LConn1 -- Transform Sensor/RConn3
  Transform Sensor/RConn2 -- PS-Simulink Converter/LConn1
  Transform Sensor/LConn1 -- G_bR/RConn1
  Transform Sensor/RConn1 -- Car_CoM/RConn1

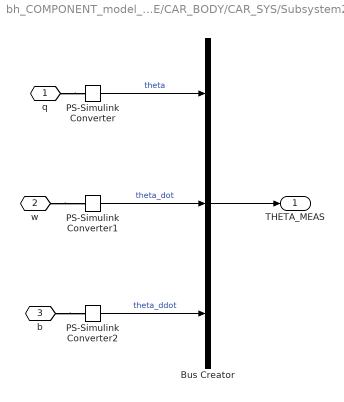
== system bh_COMPONENT_model_7dof_car_SCAPE/CAR_BODY/CAR_SYS/Subsystem2 ==
  Bus Creator : BusCreator  Inputs=3
  PS-Simulink Converter : nesl_utility/PS-Simulink Converter  PhysicalDomain=network_engine_domain  SubClassName=ps_output  LeftPortType=input  RightPortType=output  PseudoPeriodic=off  Frequencies=[]  VectorFormat=1-D array  Unit=rad  AffineConversion=off
  PS-Simulink Converter1 : nesl_utility/PS-Simulink Converter  PhysicalDomain=network_engine_domain  SubClassName=ps_output  LeftPortType=input  RightPortType=output  PseudoPeriodic=off  Frequencies=[]  VectorFormat=1-D array  Unit=rad/s  AffineConversion=off
  PS-Simulink Converter2 : nesl_utility/PS-Simulink Converter  PhysicalDomain=network_engine_domain  SubClassName=ps_output  LeftPortType=input  RightPortType=output  PseudoPeriodic=off  Frequencies=[]  VectorFormat=1-D array  Unit=rad/s^2  AffineConversion=off
  q : PMIOPort  Side=Left
  w : PMIOPort  Port=2  Side=Left
  b : PMIOPort  Port=3  Side=Left
  THETA_MEAS : Outport
  wires:
  PS-Simulink Converter2/1 -> Bus Creator/3  "theta_ddot"
  PS-Simulink Converter1/1 -> Bus Creator/2  "theta_dot"
  Bus Creator/1 -> THETA_MEAS/1
  PS-Simulink Converter/1 -> Bus Creator/1  "theta"
  connections:
  b/RConn1 -- PS-Simulink Converter2/LConn1
  w/RConn1 -- PS-Simulink Converter1/LConn1
  q/RConn1 -- PS-Simulink Converter/LConn1

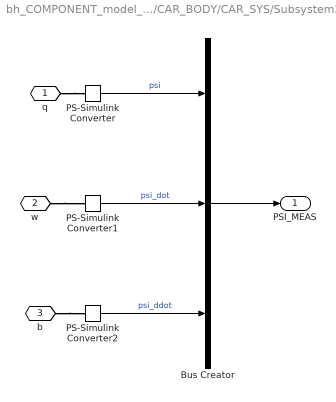
== system bh_COMPONENT_model_7dof_car_SCAPE/CAR_BODY/CAR_SYS/Subsystem3 ==
  Bus Creator : BusCreator  Inputs=3
  PS-Simulink Converter : nesl_utility/PS-Simulink Converter  PhysicalDomain=network_engine_domain  SubClassName=ps_output  LeftPortType=input  RightPortType=output  PseudoPeriodic=off  Frequencies=[]  VectorFormat=1-D array  Unit=rad  AffineConversion=off
  PS-Simulink Converter1 : nesl_utility/PS-Simulink Converter  PhysicalDomain=network_engine_domain  SubClassName=ps_output  LeftPortType=input  RightPortType=output  PseudoPeriodic=off  Frequencies=[]  VectorFormat=1-D array  Unit=rad/s  AffineConversion=off
  PS-Simulink Converter2 : nesl_utility/PS-Simulink Converter  PhysicalDomain=network_engine_domain  SubClassName=ps_output  LeftPortType=input  RightPortType=output  PseudoPeriodic=off  Frequencies=[]  VectorFormat=1-D array  Unit=rad/s^2  AffineConversion=off
  q : PMIOPort  Side=Left
  w : PMIOPort  Port=2  Side=Left
  b : PMIOPort  Port=3  Side=Left
  PSI_MEAS : Outport
  wires:
  PS-Simulink Converter2/1 -> Bus Creator/3  "psi_ddot"
  PS-Simulink Converter1/1 -> Bus Creator/2  "psi_dot"
  Bus Creator/1 -> PSI_MEAS/1
  PS-Simulink Converter/1 -> Bus Creator/1  "psi"
  connections:
  b/RConn1 -- PS-Simulink Converter2/LConn1
  w/RConn1 -- PS-Simulink Converter1/LConn1
  q/RConn1 -- PS-Simulink Converter/LConn1
